simulink model "Ex_2"  (R2020a)
settings: Solver=VariableStepAuto  StartTime=0.0  StopTime=tstop  RelTol=1e-3
values from neighbouring files (symbols this model uses):
  C = 1000e-6    (= 0.001)    [m2.m]
  L = 0.1    [m2.m]    (also in m3.m = 0.04)
  Rs = 50    [m2.m]
  tdealy = 0.05    [m2.m]
  vS = 100    [m2.m]
settings Model: Creator=abhin  LastModifiedBy=abhin

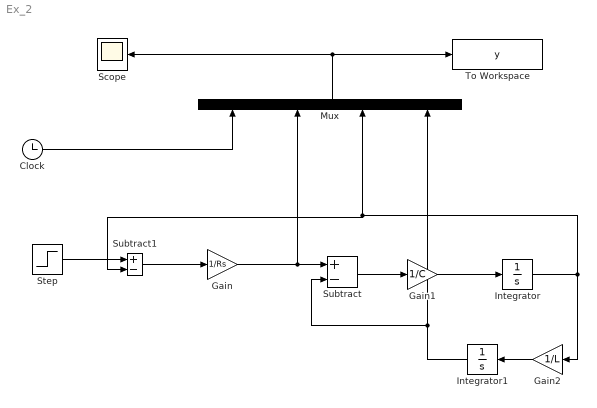
== system Ex_2 ==
  Clock : Clock
  Gain : Gain  Gain=1/Rs
  Gain1 : Gain  Gain=1/C
  Gain2 : Gain  Gain=1/L
  Integrator : Integrator
  Integrator1 : Integrator
  Mux : Mux
  Scope : Scope
  Step : Step  Time=tdealy  After=vS  SampleTime=1e-6
  Subtract : Sum  Inputs=+-
  Subtract1 : Sum  Inputs=+-
  To Workspace : ToWorkspace  VariableName=y  SaveFormat=Structure  SampleTime=-1
      settings: Save2DSignal=2-D array (concatenate along first dimension)
  wires:
  Clock/1 -> Mux/1
  Gain2/1 -> Integrator1/1
  Gain1/1 -> Integrator/1
  Mux/1 -> To Workspace/1, Scope/1
  Step/1 -> Subtract1/1
  Subtract1/1 -> Gain/1
  Gain/1 -> Mux/2, Subtract/1
  Integrator1/1 -> Subtract/2, Mux/4
  Subtract/1 -> Gain1/1
  Integrator/1 -> Gain2/1, Mux/3, Subtract1/2
